simulink model "PID_s"  (R2023a)
settings: Solver=VariableStepAuto  StartTime=0.0  StopTime=10.0  RelTol=1e-3
undefined symbols (not defined in the file): bnd_Ta_max, bnd_v_bp, DiscIntNeverNeededParam, Kaw, Kd, Ki, Kp, T_filt, Ts_ctrl
settings Model: Creator=Tan_Tram  LastModifiedBy=Tan_Tram

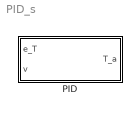
== system PID_s ==
  PID : Subsystem

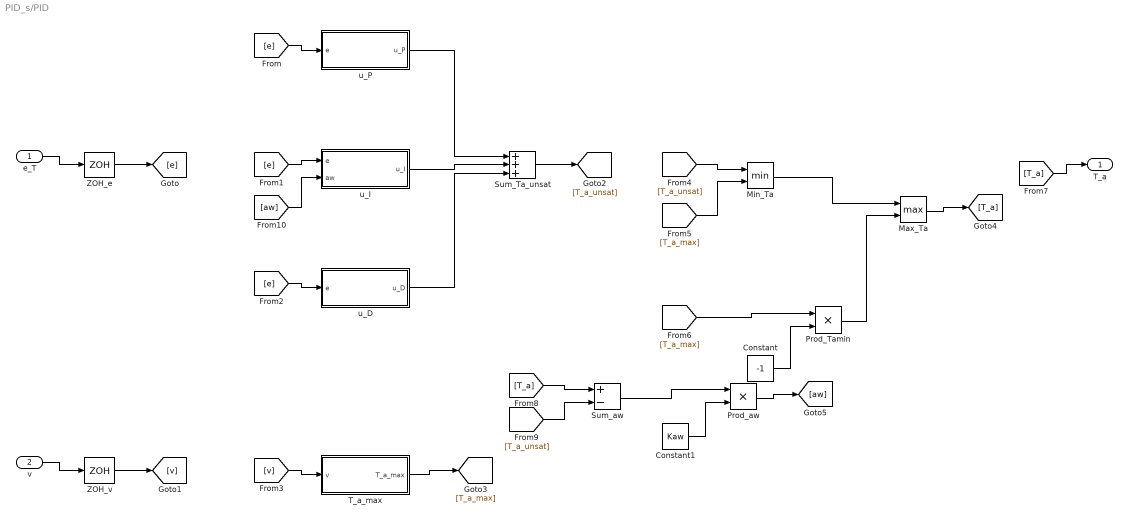
== system PID_s/PID ==
  e_T : Inport
  v : Inport  Port=2
  Constant : Constant  Value=-1
  Constant1 : Constant  Value=Kaw
  Max_Ta : MinMax  Function=max  Inputs=2
  Min_Ta : MinMax  Inputs=2
  Prod_Tamin : Product  Inputs=**
  Prod_aw : Product  Inputs=**
  Sum_Ta_unsat : Sum  Inputs=+++
  Sum_aw : Sum  Inputs=+-
  T_a_max : Subsystem
  ZOH_e : ZeroOrderHold  SampleTime=Ts_ctrl
  ZOH_v : ZeroOrderHold  SampleTime=Ts_ctrl
  u_D : Subsystem
  u_I : Subsystem
  u_P : Subsystem
  T_a : Outport
  wires:
  e_T/1 -> ZOH_e/1
  ZOH_e/1 -> [e]
  v/1 -> ZOH_v/1
  ZOH_v/1 -> [v]
  [e] -> u_P/1(e)
  [e] -> u_I/1(e)
  [e] -> u_D/1(e)
  u_P/1(u_P) -> Sum_Ta_unsat/1
  u_I/1(u_I) -> Sum_Ta_unsat/2
  u_D/1(u_D) -> Sum_Ta_unsat/3
  Sum_Ta_unsat/1 -> [T_a_unsat]
  [v] -> T_a_max/1(v)
  T_a_max/1(T_a_max) -> [T_a_max]
  [T_a_unsat] -> Min_Ta/1
  [T_a_max] -> Min_Ta/2
  [T_a_max] -> Prod_Tamin/1
  Constant/1 -> Prod_Tamin/2
  Min_Ta/1 -> Max_Ta/1
  Prod_Tamin/1 -> Max_Ta/2
  Max_Ta/1 -> [T_a]
  [T_a] -> T_a/1
  [T_a] -> Sum_aw/1
  [T_a_unsat] -> Sum_aw/2
  Sum_aw/1 -> Prod_aw/1
  Constant1/1 -> Prod_aw/2
  Prod_aw/1 -> [aw]
  [aw] -> u_I/2(aw)

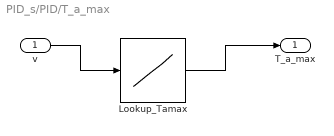
== system PID_s/PID/T_a_max ==
  v : Inport
  Lookup_Tamax : Lookup_n-D  NumberOfTableDimensions=1  BreakpointsForDimension1=bnd_v_bp  BreakpointsForDimension3=[5, 7]  Table=bnd_Ta_max  ExtrapMethod=Clip  InternalRulePriority=Speed  RndMeth=Simplest
  T_a_max : Outport
  wires:
  v/1 -> Lookup_Tamax/1
  Lookup_Tamax/1 -> T_a_max/1

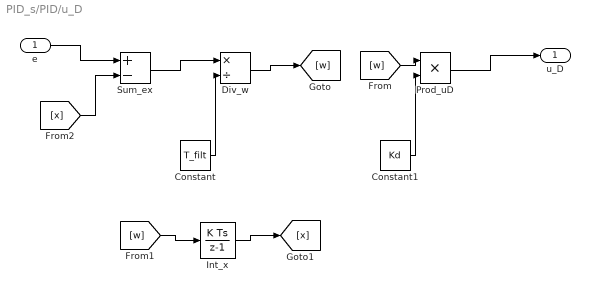
== system PID_s/PID/u_D ==
  e : Inport
  Constant : Constant  Value=T_filt
  Constant1 : Constant  Value=Kd
  Div_w : Product  Inputs=*/
  Int_x : DiscreteIntegrator  SampleTime=Ts_ctrl  ICPrevOutput=DiscIntNeverNeededParam  ICPrevScaledInput=DiscIntNeverNeededParam
  Prod_uD : Product  Inputs=**
  Sum_ex : Sum  Inputs=+-
  u_D : Outport
  wires:
  Div_w/1 -> [w]
  e/1 -> Sum_ex/1
  [x] -> Sum_ex/2
  Sum_ex/1 -> Div_w/1
  Constant/1 -> Div_w/2
  [w] -> Prod_uD/1
  Constant1/1 -> Prod_uD/2
  Prod_uD/1 -> u_D/1
  [w] -> Int_x/1
  Int_x/1 -> [x]

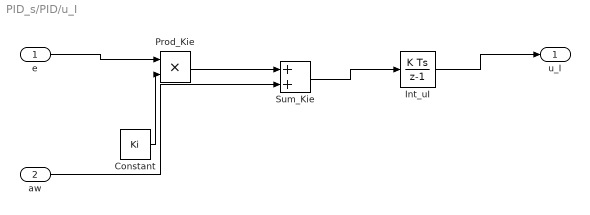
== system PID_s/PID/u_I ==
  e : Inport
  aw : Inport  Port=2
  Constant : Constant  Value=Ki
  Int_uI : DiscreteIntegrator  SampleTime=Ts_ctrl  ICPrevOutput=DiscIntNeverNeededParam  ICPrevScaledInput=DiscIntNeverNeededParam
  Prod_Kie : Product  Inputs=**
  Sum_Kie : Sum
  u_I : Outport
  wires:
  e/1 -> Prod_Kie/1
  Constant/1 -> Prod_Kie/2
  Prod_Kie/1 -> Sum_Kie/1
  aw/1 -> Sum_Kie/2
  Sum_Kie/1 -> Int_uI/1
  Int_uI/1 -> u_I/1

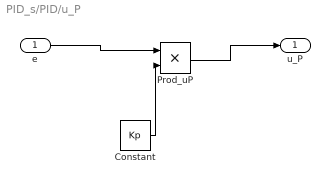
== system PID_s/PID/u_P ==
  e : Inport
  Constant : Constant  Value=Kp
  Prod_uP : Product  Inputs=**
  u_P : Outport
  wires:
  e/1 -> Prod_uP/1
  Constant/1 -> Prod_uP/2
  Prod_uP/1 -> u_P/1
